simulink model "TorqueVect"  (R2022a)
settings: Solver=VariableStepAuto  StartTime=0.0  StopTime=32  RelTol=1e-3
PreLoadFcn:
  | run('Parameters\FSE_Parameters.m')
undefined symbols (not defined in the file): BRegenEnabledButton, canChannel, CyalphaLookUp, efficiency, Fz_curve, Fz_scaling_long, gearR, izz, jw, Kd, kd, Ki, ki, Kp, kp, l_f, l_r, lambda, m, Mz_max, N, N_lat, N_long, P_max, pid_kd_lat, pid_kd_long, pid_ki_lat, pid_ki_long, pid_kp_lat, pid_kp_long, R_max, rw, steerR, T_i_max, TC_Decr_Gas, TC_Derivative, TC_Incr_Gas, TC_On, TC_Relay_Off, TC_Relay_On, tireCornerStiffness, Ts, TV_On, TV_Override, velocity_lookup, velocity_lookup_lat, y_ref, yrr_scaling
libraries: simulink x218, slpidlib x135, CarMaker4SL x101, TractionControlLibrary x13, canmsglib x9, canlib x8, TorqueVectoringLibrary x6, simulink_extras x4, PedalConversionLibrary x3, PowerControlLibrary x1
(part 18 of 26)

== system TorqueVect/CarMaker/IPG Vehicle/PowerTrain/PTControl Example/PTControl_ALL_CTRL_VC_REGEN/Subsystem1/PowerControl1/PID ==
  PError : Inport
  P_PC : Inport  Port=2
  D_PC : Inport  Port=3
  I_PC : Inport  Port=4
  ResetPID_PC : Inport  Port=5
  PID Controller : slpidlib/PID Controller  Controller=PID  Form=Parallel  TimeDomain=Discrete-time  UseExternalTs=off  SampleTime=0.005  IntegratorMethod=Backward Euler  FilterMethod=Forward Euler  ControllerParametersSource=external  P=1  I=1  UseKiTs=on  D=0  N=100  UseFilter=off  TunerSelectOption=Transfer Function Based (PID Tuner App)  InitialConditionSource=internal  InitialConditionForIntegrator=0  InitialConditionForFilter=0  DifferentiatorICPrevScaledInput=0  ExternalReset=rising  TrackingMode=off  Kt=1  LimitOutput=on  SatLimitsSource=internal  UpperSaturationLimit=80000  LowerSaturationLimit=0  LinearizeAsGain=on  AntiWindupMode=clamping  Kb=2  SaturateOnIntegerOverflow=on  POutMin=[]  POutMax=[]  IOutMin=[]  IOutMax=[]  DOutMin=[]  DOutMax=[]  NOutMin=[]  NOutMax=[]  SumOutMin=[]  SumOutMax=[]  SaturationOutMin=[]  SaturationOutMax=[]  PParamMin=[]  PParamMax=[]  IParamMin=[]  IParamMax=[]  DParamMin=[]  DParamMax=[]  NParamMin=[]  NParamMax=[]  KbParamMin=[]  KbParamMax=[]  KtParamMin=[]  KtParamMax=[]  KbOutMin=[]  KbOutMax=[]  KtOutMin=[]  KtOutMax=[]  IntegratorOutMin=[]  IntegratorOutMax=[]  FilterOutMin=[]  FilterOutMax=[]  SumI1OutMin=[]  SumI1OutMax=[]  SumI2OutMin=[]  SumI2OutMax=[]  SumI3OutMin=[]  SumI3OutMax=[]  SumI4OutMin=[]  SumI4OutMax=[]  SumDOutMin=[]  SumDOutMax=[]  DifferentiatorOutMin=[]  DifferentiatorOutMax=[]  FilterDiffOutCoefMin=[]  FilterDiffOutCoefMax=[]  ReciprocalOutMin=[]  ReciprocalOutMax=[]  SumDenOutMin=[]  SumDenOutMax=[]  SumNumOutMin=[]  SumNumOutMax=[]  DivideOutMin=[]  DivideOutMax=[]  UdiffTsProdOutMin=[]  UdiffTsProdOutMax=[]  NTsProdOutMin=[]  NTsProdOutMax=[]  UintegralTsProdOutMin=[]  UintegralTsProdOutMax=[]  UngainTsProdOutMin=[]  UngainTsProdOutMax=[]  ClampingZeroOutDataTypeStr=Inherit: Inherit via back propagation  ClampingZeroOutMin=[]  ClampingZeroOutMax=[]  FilterDenConstantOutDataTypeStr=Inherit: Inherit via back propagation  FilterDenConstantOutMin=[]  FilterDenConstantOutMax=[]  PCopyOutDataTypeStr=Inherit: Inherit via back propagation  PCopyOutMin=[]  PCopyOutMax=[]  NCopyOutDataTypeStr=Inherit: Inherit via back propagation  NCopyOutMin=[]  NCopyOutMax=[]  IntegratorContinuousStateAttributes=''  IntegratorStateMustResolveToSignalObject=off  IntegratorRTWStateStorageClass=Auto  FilterContinuousStateAttributes=''  FilterStateMustResolveToSignalObject=off  FilterRTWStateStorageClass=Auto  ParallelPVariant=ExternalParameters  IdealPVariant=Disabled  IVariant=ExternalParameters  DVariant=ExternalParameters  IntegratorVariant=Discrete  SatVariant=Enabled  AWVariant=DiscClampingParallel  PCopyVariant=Disabled  TRVariant=Disabled  FdbkBlocksVariant=Feedback  IdealPFdbkVariant=Passthrough  SatFdbkVariant=Passthrough  DerivativeFilterVariant=Differentiator  NVariant=Passthrough  NCopyVariant=Disabled_SignalSpec  FilterICVariant=InternalICsDifferentiator  IntegratorICVariant=InternalICs  ExternalResetVariant=ExternalReset  TRSumVariant=Passthrough  SumFdbkVariant=Enabled  SumVariant=Sum_PID  TsampFilterVariant=InternalTs  TsampNgainVariant=Passthrough  TsampIntegralVariant=Passthrough  ExternalSaturationOutDataTypeStr=Inherit: Same as second input  aMode=0
  PReductionTotal : Outport
  wires:
  PID Controller/1 -> PReductionTotal/1  "control input delta_P"
  D_PC/1 -> PID Controller/4
  P_PC/1 -> PID Controller/2
  PError/1 -> PID Controller/1
  I_PC/1 -> PID Controller/3
  ResetPID_PC/1 -> PID Controller/5

== system TorqueVect/CarMaker/IPG Vehicle/PowerTrain/PTControl Example/PTControl_ALL_CTRL_VC_REGEN/Subsystem1/PowerControl1/PowerError ==
  PPositiveTotal : Inport  Unit=W  PortDimensions=1
      settings: AttributesFormatString=%<Unit>
  FF_PC : Inport  Port=2
  PLimit : Inport  Port=3  OutMin=0  OutMax=80000  Unit=W  PortDimensions=1
      settings: AttributesFormatString=[%<OutMin>, %<OutMax>] %<Unit>
  Product5 : Product
  Saturation2 : Saturate  UpperLimit=250000  LowerLimit=0
      settings: AttributesFormatString=[%<LowerLimit>, %<UpperLimit>] W
  Subtract2 : Sum  Inputs=+-
  PError : Outport  Unit=W  PortDimensions=1
      settings: AttributesFormatString=%<Unit>
  wires:
  FF_PC/1 -> Product5/2
  Subtract2/1 -> Saturation2/1
  PLimit/1 -> Subtract2/2
  PPositiveTotal/1 -> Product5/1
  Saturation2/1 -> PError/1  "power error"
  Product5/1 -> Subtract2/1

== system TorqueVect/CarMaker/IPG Vehicle/PowerTrain/PTControl Example/PTControl_ALL_CTRL_VC_REGEN/Subsystem1/PowerControl1/ResetPID_PC ==
  rThrottlePedal : Inport
  PReductionTotal : Inport  Port=2
  AND : Logic  IconShape=distinctive  AllPortsSameDT=off  OutDataTypeStr=boolean
  AND1 : Logic  Inputs=3  IconShape=distinctive  AllPortsSameDT=off  OutDataTypeStr=boolean
  Compare To Constant1 : simulink/Logic and Bit Operations/Compare To Constant  relop=<=  const=0.1  OutDataTypeStr=boolean
  Compare To Constant2 : simulink/Logic and Bit Operations/Compare To Constant  relop=<=  const=0.15  OutDataTypeStr=boolean
  Compare To Constant3 : simulink/Logic and Bit Operations/Compare To Constant  relop=>=  const=0.09  OutDataTypeStr=boolean
  Compare To Constant4 : simulink/Logic and Bit Operations/Compare To Constant  relop=>  const=0  OutDataTypeStr=boolean
  Detect Fall Negative1 : simulink/Logic and Bit Operations/Detect Fall Negative  vinit=0  OutDataTypeStr=boolean
      settings: SourceProductBaseCode=SL
  Discrete Derivative1 : simulink/Discrete/Discrete Derivative  gainval=1.0  ICPrevScaledInput=0.0  OutMin=[]  OutMax=[]  OutDataType=fixdt(1, 16)  OutScaling=2^-10  DoSatur=off
  OR : Logic  Operator=OR  IconShape=distinctive  AllPortsSameDT=off  OutDataTypeStr=boolean
  ResetPID_PC : Outport
  wires:
  rThrottlePedal/1 -> Compare To Constant1/1, Compare To Constant3/1, Compare To Constant2/1, Discrete Derivative1/1
  Discrete Derivative1/1 -> Detect Fall Negative1/1
  Detect Fall Negative1/1 -> AND1/2  "accel_pedal_falling_or"
  Compare To Constant2/1 -> AND1/1
  Compare To Constant3/1 -> AND1/3
  OR/1 -> ResetPID_PC/1
  AND1/1 -> OR/1
  AND/1 -> OR/2
  Compare To Constant1/1 -> AND/1
  Compare To Constant4/1 -> AND/2
  PReductionTotal/1 -> Compare To Constant4/1

== system TorqueVect/CarMaker/IPG Vehicle/PowerTrain/PTControl Example/PTControl_ALL_CTRL_VC_REGEN/Subsystem1/PowerControl1/Subsystem ==
  PReductionTotal : Inport
  rSplitF : Inport  Port=2
  Product : Product
  Sum : Sum  Inputs=|+-
  PReductionR : Outport
  PReductionF : Outport  Port=2
  wires:
  rSplitF/1 -> Product/2
  PReductionTotal/1 -> Sum/1, Product/1
  Product/1 -> PReductionF/1, Sum/2
  Sum/1 -> PReductionR/1

== system TorqueVect/CarMaker/IPG Vehicle/PowerTrain/PTControl Example/PTControl_ALL_CTRL_VC_REGEN/Subsystem1/PowerControl1/TotalPower ==
  MMotorFL : Inport  OutMin=-42  OutMax=42  Unit=N*m  PortDimensions=1
      settings: AttributesFormatString=[%<OutMin>, %<OutMax>] %<Unit>
  nMotorFL : Inport  Port=2  OutMin=-3000  OutMax=3000  Unit=rad/s  PortDimensions=1
      settings: AttributesFormatString=[%<OutMin>, %<OutMax>] %<Unit>
  MMotorFR : Inport  Port=3  OutMin=-42  OutMax=42  Unit=N*m  PortDimensions=1
      settings: AttributesFormatString=[%<OutMin>, %<OutMax>] %<Unit>
  nMotorFR : Inport  Port=4  OutMin=-3000  OutMax=3000  Unit=rad/s  PortDimensions=1
      settings: AttributesFormatString=[%<OutMin>, %<OutMax>] %<Unit>
  MMotorRL : Inport  Port=5  OutMin=-42  OutMax=42  Unit=N*m  PortDimensions=1
      settings: AttributesFormatString=[%<OutMin>, %<OutMax>] %<Unit>
  nMotorRL : Inport  Port=6  OutMin=-3000  OutMax=3000  Unit=rad/s  PortDimensions=1
      settings: AttributesFormatString=[%<OutMin>, %<OutMax>] %<Unit>
  MMotorRR : Inport  Port=7  OutMin=-42  OutMax=42  Unit=N*m  PortDimensions=1
      settings: AttributesFormatString=[%<OutMin>, %<OutMax>] %<Unit>
  nMotorRR : Inport  Port=8  OutMin=-3000  OutMax=3000  Unit=rad/s  PortDimensions=1
      settings: AttributesFormatString=[%<OutMin>, %<OutMax>] %<Unit>
  PMeasured : Inport  Port=9  OutMin=-250000  OutMax=250000  Unit=W  PortDimensions=1
      settings: AttributesFormatString=[%<OutMin>, %<OutMax>] %<Unit>
  BMeasuredEnable : Inport  Port=10  OutMin=0  OutMax=1  PortDimensions=1
      settings: AttributesFormatString=[%<OutMin> / %<OutMax>]
  Product{2,7..9} (4 alike) : Product
  Saturation{1,3..5} (4 alike) : Saturate  UpperLimit=250000  LowerLimit=0
  Sum1 : Sum  Inputs=++++
  Sum3 : Sum  Inputs=++++
  Switch : Switch  Threshold=1  SaturateOnIntegerOverflow=off  InputSameDT=off
  Switch3 : Switch  Threshold=1  SaturateOnIntegerOverflow=off  InputSameDT=off
  Terminator : Terminator
  PPositiveTotal : Outport  OutMin=0  OutMax=250000  Unit=W  PortDimensions=1
      settings: AttributesFormatString=[%<OutMin>, %<OutMax>] %<Unit>
  wires:
  MMotorRR/1 -> Product9/2
  nMotorRR/1 -> Product9/1
  nMotorRL/1 -> Product8/2
  MMotorRL/1 -> Product8/1
  nMotorFR/1 -> Product7/2
  MMotorFR/1 -> Product7/1
  nMotorFL/1 -> Product2/2
  MMotorFL/1 -> Product2/1
  Product9/1 -> Saturation5/1, Sum1/4
  Product8/1 -> Saturation4/1, Sum1/3
  Product7/1 -> Saturation3/1, Sum1/2
  BMeasuredEnable/1 -> Switch/2, Switch3/2
  Switch3/1 -> Terminator/1
  PMeasured/1 -> Switch/1, Switch3/1
  Switch/1 -> PPositiveTotal/1
  Sum1/1 -> Switch3/3  "tot_powerrrr_RC"
  Saturation1/1 -> Sum3/1
  Saturation4/1 -> Sum3/3
  Product2/1 -> Saturation1/1, Sum1/1
  Saturation5/1 -> Sum3/4
  Sum3/1 -> Switch/3  "tot_powerrrr_PC"
  Saturation3/1 -> Sum3/2

== system TorqueVect/CarMaker/IPG Vehicle/PowerTrain/PTControl Example/PTControl_ALL_CTRL_VC_REGEN/Subsystem1/PowerControl1/WheelTorqueOut ==
  PReductionF : Inport
  PReductionR : Inport  Port=2
  nMotorFL : Inport  Port=3
  nMotorFR : Inport  Port=4
  nMotorRL : Inport  Port=5
  nMotorRR : Inport  Port=6
  Divide{1..4} (4 alike) : Product  Inputs=*/
  Gain : Gain  Gain=0.5
  Gain1 : Gain  Gain=0.5
  Saturation{,5..7} (4 alike) : Saturate  UpperLimit=42  LowerLimit=-42
  Saturation{1..4} (4 alike) : Saturate  UpperLimit=30000  LowerLimit=eps
  MReductionMotorFL : Outport
  MReductionMotorFR : Outport  Port=2
  MReductionMotorRL : Outport  Port=3
  MReductionMotorRR : Outport  Port=4
  wires:
  Divide4/1 -> Saturation7/1
  Divide3/1 -> Saturation6/1
  Divide2/1 -> Saturation5/1
  Divide1/1 -> Saturation/1
  Saturation4/1 -> Divide4/2
  Saturation3/1 -> Divide3/2
  nMotorRR/1 -> Saturation4/1
  nMotorRL/1 -> Saturation3/1
  Gain1/1 -> Divide3/1, Divide4/1
  Saturation2/1 -> Divide2/2
  Saturation1/1 -> Divide1/2
  nMotorFR/1 -> Saturation2/1
  nMotorFL/1 -> Saturation1/1
  Gain/1 -> Divide1/1, Divide2/1
  PReductionR/1 -> Gain1/1
  PReductionF/1 -> Gain/1
  Saturation/1 -> MReductionMotorFL/1
  Saturation5/1 -> MReductionMotorFR/1
  Saturation6/1 -> MReductionMotorRL/1
  Saturation7/1 -> MReductionMotorRR/1

== system TorqueVect/CarMaker/IPG Vehicle/PowerTrain/PTControl Example/PTControl_ALL_CTRL_VC_REGEN/Subsystem1/TC/Slip Ratio Measurement ==
  vLong1 : Inport  Unit=m/s
      settings: AttributesFormatString=%<Unit>
  nMotorFL : Inport  Port=2  Unit=rad/s  PortDimensions=1
      settings: AttributesFormatString=%<Unit>
  nMotorFR : Inport  Port=3  Unit=rad/s  PortDimensions=1
      settings: AttributesFormatString=%<Unit>
  nMotorRL : Inport  Port=4  Unit=rad/s  PortDimensions=1
      settings: AttributesFormatString=%<Unit>
  nMotorRR : Inport  Port=5  Unit=rad/s  PortDimensions=1
      settings: AttributesFormatString=%<Unit>
  aSteerFL : Inport  Port=6
  aSteerFR : Inport  Port=7
  nYaw : Inport  Port=8
  Add : Sum  Inputs=+-
  Add1 : Sum
  Add2 : Sum  Inputs=-+
  Constant : Constant  Value=[0 0 0 0]
  Constant3 : Constant
  Cos : Trigonometry  Operator=cos
  Cos1 : Trigonometry  Operator=cos
  Demux : Demux
  Demux1 : Demux
  Divide : Product  Inputs=/*
  Divide1 : Product  Inputs=*/
  Divide2 : Product  Inputs=/*
  Gain : Gain  Gain=0.1975/13.39
  Mux : Mux
  Mux1 : Mux
  Product : Product
  Saturation : Saturate  UpperLimit=60  LowerLimit=eps
  Saturation1 : Saturate  UpperLimit=1  LowerLimit=0
  Switch1 : Switch  Criteria=u2 > Threshold  Threshold=0.25  SaturateOnIntegerOverflow=off  InputSameDT=off
  halfTrackWidth : Constant  Value=0.5588
  vLong1_1 : InportShadow  Unit=m/s
      settings: AttributesFormatString=%<Unit>
  rSlipMeasuredFL : Outport
  rSlipMeasuredFR : Outport  Port=2
  rSlipMeasuredRL : Outport  Port=3
  rSlipMeasuredRR : Outport  Port=4
  debug : Outport  Port=5
  wires:
  vLong1_1/1 -> Switch1/2
  Add/1 -> Mux1/3, Divide/2  "vWheelFromCarLongRL"
  nMotorFR/1 -> Mux/2
  halfTrackWidth/1 -> Product/2
  Mux1/1 -> Saturation/1
  vLong1/1 -> Add/1, Add1/1
  Demux1/4 -> rSlipMeasuredRR/1
  nYaw/1 -> Product/1
  Saturation1/1 -> Demux1/1
  nMotorRL/1 -> Mux/3
  Demux1/3 -> rSlipMeasuredRL/1
  Gain/1 -> Divide2/2  "m/s"
  Product/1 -> Add1/2, Add/2
  Add1/1 -> Mux1/4, Divide1/1  "vWheelFromCarLongRR"
  nMotorFL/1 -> Mux/1
  Saturation/1 -> Divide2/1
  Cos1/1 -> Divide1/2
  nMotorRR/1 -> Mux/4
  Divide1/1 -> Mux1/2  "vWheelFromCarLongFR"
  Demux1/1 -> rSlipMeasuredFL/1
  Mux/1 -> Gain/1  "omega"
  Switch1/1 -> Saturation1/1
  Cos/1 -> Divide/1
  Constant/1 -> Switch1/3
  Divide/1 -> Mux1/1  "vWheelFromCarLongFL"
  Demux1/2 -> rSlipMeasuredFR/1
  aSteerFR/1 -> Cos1/1
  aSteerFL/1 -> Cos/1
  Divide2/1 -> Add2/2
  Constant3/1 -> Add2/1
  Add2/1 -> Demux/1, Switch1/1
  Demux/1 -> debug/1

== system TorqueVect/CarMaker/IPG Vehicle/PowerTrain/PTControl Example/PTControl_ALL_CTRL_VC_REGEN/Subsystem1/TC/TractionControlFL ==
  rSlipTarget : Inport
  rSlipMeasured : Inport  Port=2
  BEnableTC : Inport  Port=3
  P_TC : Inport  Port=4
  D_TC : Inport  Port=5
  I_TC : Inport  Port=6
  FF_TC : Inport  Port=7
  MMotorMax : Inport  Port=8
  MMotorRequest : Inport  Port=9
  resetTC : Inport  Port=10
  If : If  NumInputs=2  IfExpression=u1 <= 0  ElseIfExpressions=u2 > u1
  If Action Subsystem : Subsystem  TreatAsAtomicUnit=on
  If Action Subsystem1 : Subsystem  TreatAsAtomicUnit=on
  If Action Subsystem2 : Subsystem  TreatAsAtomicUnit=on
  Merge : Merge  Inputs=3
  PID Controller : Subsystem  TreatAsAtomicUnit=on
  Product : Product
  Product1 : Product
  Saturation : Saturate  UpperLimit=1  LowerLimit=0
  Saturation1 : Saturate  UpperLimit=21  LowerLimit=0
  Sum1 : Sum  Inputs=|-+
  MMotorDemanded : Outport  VectorParamsAs1DForOutWhenUnconnected=off
  wires:
  rSlipTarget/1 -> Sum1/1
  MMotorRequest/1 -> If Action Subsystem/1(MMotorRequest), If/1, If Action Subsystem2/1(MMotorRequest)
  Saturation1/1 -> If Action Subsystem2/2(In2), If/2
  If/2 -> If Action Subsystem1/Action
  P_TC/1 -> PID Controller/3(Kp_TC)
  If Action Subsystem2/1(Out1) -> Merge/3
  FF_TC/1 -> Product/2
  Product/1 -> Sum1/2
  D_TC/1 -> PID Controller/4(Kd_TC)
  Saturation/1 -> PID Controller/1(rSlipError)
  If Action Subsystem/1(Out1) -> Merge/1
  Product1/1 -> Saturation/1
  If/3 -> If Action Subsystem2/Action
  BEnableTC/1 -> Product1/2, PID Controller/2(BEnable_TC)
  If Action Subsystem1/1(Out1) -> Merge/2
  PID Controller/1(MMotorReduction) -> Saturation1/1
  I_TC/1 -> PID Controller/5(Ki_TC)
  Merge/1 -> MMotorDemanded/1
  Sum1/1 -> Product1/1
  If/1 -> If Action Subsystem/Action
  rSlipMeasured/1 -> Product/1
  MMotorMax/1 -> PID Controller/6(MMotorMax)
  resetTC/1 -> PID Controller/7(resetTC)

== system TorqueVect/CarMaker/IPG Vehicle/PowerTrain/PTControl Example/PTControl_ALL_CTRL_VC_REGEN/Subsystem1/TC/TractionControlFR ==
  rSlipTarget : Inport
  rSlipMeasured : Inport  Port=2
  BEnableTC : Inport  Port=3
  P_TC : Inport  Port=4
  D_TC : Inport  Port=5
  I_TC : Inport  Port=6
  FF_TC : Inport  Port=7
  MMotorMax : Inport  Port=8
  MMotorRequest : Inport  Port=9
  resetTC : Inport  Port=10
  If : If  NumInputs=2  IfExpression=u1 <= 0  ElseIfExpressions=u2 > u1
  If Action Subsystem : Subsystem  TreatAsAtomicUnit=on
  If Action Subsystem1 : Subsystem  TreatAsAtomicUnit=on
  If Action Subsystem2 : Subsystem  TreatAsAtomicUnit=on
  Merge : Merge  Inputs=3
  PID Controller : Subsystem  TreatAsAtomicUnit=on
  Product : Product
  Product1 : Product
  Saturation : Saturate  UpperLimit=1  LowerLimit=0
  Saturation1 : Saturate  UpperLimit=21  LowerLimit=0
  Sum1 : Sum  Inputs=|-+
  MMotorDemanded : Outport  VectorParamsAs1DForOutWhenUnconnected=off
  wires:
  rSlipTarget/1 -> Sum1/1
  MMotorRequest/1 -> If Action Subsystem/1(MMotorRequest), If/1, If Action Subsystem2/1(MMotorRequest)
  Saturation1/1 -> If Action Subsystem2/2(In2), If/2
  If/2 -> If Action Subsystem1/Action
  P_TC/1 -> PID Controller/3(Kp_TC)
  If Action Subsystem2/1(Out1) -> Merge/3
  FF_TC/1 -> Product/2
  Product/1 -> Sum1/2
  D_TC/1 -> PID Controller/4(Kd_TC)
  Saturation/1 -> PID Controller/1(rSlipError)
  If Action Subsystem/1(Out1) -> Merge/1
  Product1/1 -> Saturation/1
  If/3 -> If Action Subsystem2/Action
  BEnableTC/1 -> Product1/2, PID Controller/2(BEnable_TC)
  If Action Subsystem1/1(Out1) -> Merge/2
  PID Controller/1(MMotorReduction) -> Saturation1/1
  I_TC/1 -> PID Controller/5(Ki_TC)
  Merge/1 -> MMotorDemanded/1
  Sum1/1 -> Product1/1
  If/1 -> If Action Subsystem/Action
  rSlipMeasured/1 -> Product/1
  MMotorMax/1 -> PID Controller/6(MMotorMax)
  resetTC/1 -> PID Controller/7(resetTC)

== system TorqueVect/CarMaker/IPG Vehicle/PowerTrain/PTControl Example/PTControl_ALL_CTRL_VC_REGEN/Subsystem1/TC/TractionControlRL ==
  rSlipTarget : Inport
  rSlipMeasured : Inport  Port=2
  BEnableTC : Inport  Port=3
  P_TC : Inport  Port=4
  D_TC : Inport  Port=5
  I_TC : Inport  Port=6
  FF_TC : Inport  Port=7
  MMotorMax : Inport  Port=8
  MMotorRequest : Inport  Port=9
  resetTC : Inport  Port=10
  If : If  NumInputs=2  IfExpression=u1 <= 0  ElseIfExpressions=u2 > u1
  If Action Subsystem : Subsystem  TreatAsAtomicUnit=on
  If Action Subsystem1 : Subsystem  TreatAsAtomicUnit=on
  If Action Subsystem2 : Subsystem  TreatAsAtomicUnit=on
  Merge : Merge  Inputs=3
  PID Controller : Subsystem  TreatAsAtomicUnit=on
  Product : Product
  Product1 : Product
  Saturation : Saturate  UpperLimit=1  LowerLimit=0
  Saturation1 : Saturate  UpperLimit=21  LowerLimit=0
  Sum1 : Sum  Inputs=|-+
  MMotorDemanded : Outport  VectorParamsAs1DForOutWhenUnconnected=off
  wires:
  rSlipTarget/1 -> Sum1/1
  MMotorRequest/1 -> If Action Subsystem/1(MMotorRequest), If/1, If Action Subsystem2/1(MMotorRequest)
  Saturation1/1 -> If Action Subsystem2/2(In2), If/2
  If/2 -> If Action Subsystem1/Action
  P_TC/1 -> PID Controller/3(Kp_TC)
  If Action Subsystem2/1(Out1) -> Merge/3
  FF_TC/1 -> Product/2
  Product/1 -> Sum1/2
  D_TC/1 -> PID Controller/4(Kd_TC)
  Saturation/1 -> PID Controller/1(rSlipError)
  If Action Subsystem/1(Out1) -> Merge/1
  Product1/1 -> Saturation/1
  If/3 -> If Action Subsystem2/Action
  BEnableTC/1 -> Product1/2, PID Controller/2(BEnable_TC)
  If Action Subsystem1/1(Out1) -> Merge/2
  PID Controller/1(MMotorReduction) -> Saturation1/1
  I_TC/1 -> PID Controller/5(Ki_TC)
  Merge/1 -> MMotorDemanded/1
  Sum1/1 -> Product1/1
  If/1 -> If Action Subsystem/Action
  rSlipMeasured/1 -> Product/1
  MMotorMax/1 -> PID Controller/6(MMotorMax)
  resetTC/1 -> PID Controller/7(resetTC)

== system TorqueVect/CarMaker/IPG Vehicle/PowerTrain/PTControl Example/PTControl_ALL_CTRL_VC_REGEN/Subsystem1/TC/TractionControlRR ==
  rSlipTarget : Inport
  rSlipMeasured : Inport  Port=2
  BEnableTC : Inport  Port=3
  P_TC : Inport  Port=4
  D_TC : Inport  Port=5
  I_TC : Inport  Port=6
  FF_TC : Inport  Port=7
  MMotorMax : Inport  Port=8
  MMotorRequest : Inport  Port=9
  resetTC : Inport  Port=10
  If : If  NumInputs=2  IfExpression=u1 <= 0  ElseIfExpressions=u2 > u1
  If Action Subsystem : Subsystem  TreatAsAtomicUnit=on
  If Action Subsystem1 : Subsystem  TreatAsAtomicUnit=on
  If Action Subsystem2 : Subsystem  TreatAsAtomicUnit=on
  Merge : Merge  Inputs=3
  PID Controller : Subsystem  TreatAsAtomicUnit=on
  Product : Product
  Product1 : Product
  Saturation : Saturate  UpperLimit=1  LowerLimit=0
  Saturation1 : Saturate  UpperLimit=21  LowerLimit=0
  Sum1 : Sum  Inputs=|-+
  MMotorDemanded : Outport  VectorParamsAs1DForOutWhenUnconnected=off
  wires:
  rSlipTarget/1 -> Sum1/1
  MMotorRequest/1 -> If Action Subsystem/1(MMotorRequest), If/1, If Action Subsystem2/1(MMotorRequest)
  Saturation1/1 -> If Action Subsystem2/2(In2), If/2
  If/2 -> If Action Subsystem1/Action
  P_TC/1 -> PID Controller/3(Kp_TC)
  If Action Subsystem2/1(Out1) -> Merge/3
  FF_TC/1 -> Product/2
  Product/1 -> Sum1/2
  D_TC/1 -> PID Controller/4(Kd_TC)
  Saturation/1 -> PID Controller/1(rSlipError)
  If Action Subsystem/1(Out1) -> Merge/1
  Product1/1 -> Saturation/1
  If/3 -> If Action Subsystem2/Action
  BEnableTC/1 -> PID Controller/2(BEnable_TC), Product1/2
  If Action Subsystem1/1(Out1) -> Merge/2
  PID Controller/1(MMotorReduction) -> Saturation1/1
  I_TC/1 -> PID Controller/5(Ki_TC)
  Merge/1 -> MMotorDemanded/1
  Sum1/1 -> Product1/1
  If/1 -> If Action Subsystem/Action
  rSlipMeasured/1 -> Product/1
  MMotorMax/1 -> PID Controller/6(MMotorMax)
  resetTC/1 -> PID Controller/7(resetTC)

== system TorqueVect/CarMaker/IPG Vehicle/PowerTrain/PTControl Example/PTControl_ALL_CTRL_VC_REGEN/Subsystem1/Torque Modification/Torque Limit Check FL ==
  note: Checks for max value below 0 Nm when RC is acting
  note: Checks for min value when PC is acting
  MTorqueNewFL : Inport
  MDemandMotorFL : Inport  Port=2
  Max : MinMax  Function=max  Inputs=2
  Min : MinMax  Inputs=2
  Saturation : Saturate  UpperLimit=0  LowerLimit=-21
  Saturation1 : Saturate  UpperLimit=21  LowerLimit=0
  Switch : Switch  Criteria=u2 > Threshold  SaturateOnIntegerOverflow=off  InputSameDT=off
  MTorqueModFL : Outport
  wires:
  MDemandMotorFL/1 -> [MDemandMotorRL]
  [MDemandMotorRL] -> Min/1
  MTorqueNewFL/1 -> Saturation/1, Saturation1/1
  Switch/1 -> MTorqueModFL/1
  [MDemandMotorRL] -> Switch/2
  Min/1 -> Switch/1
  Max/1 -> Switch/3
  [MDemandMotorRL] -> Max/2
  Saturation/1 -> Max/1
  Saturation1/1 -> Min/2

== system TorqueVect/CarMaker/IPG Vehicle/PowerTrain/PTControl Example/PTControl_ALL_CTRL_VC_REGEN/Subsystem1/Torque Modification/Torque Limit Check FR ==
  note: Checks for max value below 0 Nm when RC is acting
  note: Checks for min value when PC is acting
  MTorqueNewFR : Inport
  MDemandMotorFR : Inport  Port=2
  Max : MinMax  Function=max  Inputs=2
  Min : MinMax  Inputs=2
  Saturation : Saturate  UpperLimit=0  LowerLimit=-21
  Saturation1 : Saturate  UpperLimit=21  LowerLimit=0
  Switch : Switch  Criteria=u2 > Threshold  SaturateOnIntegerOverflow=off  InputSameDT=off
  MTorqueModFR : Outport
  wires:
  MDemandMotorFR/1 -> [MDemandMotorRL]
  [MDemandMotorRL] -> Min/1
  MTorqueNewFR/1 -> Saturation/1, Saturation1/1
  Switch/1 -> MTorqueModFR/1
  [MDemandMotorRL] -> Switch/2
  Min/1 -> Switch/1
  Max/1 -> Switch/3
  [MDemandMotorRL] -> Max/2
  Saturation/1 -> Max/1
  Saturation1/1 -> Min/2

== system TorqueVect/CarMaker/IPG Vehicle/PowerTrain/PTControl Example/PTControl_ALL_CTRL_VC_REGEN/Subsystem1/Torque Modification/Torque Limit Check RL ==
  note: Checks for max value below 0 Nm when RC is acting
  note: Checks for min value when PC is acting
  MTorqueNewRL : Inport
  MDemandMotorRL : Inport  Port=2
  Max : MinMax  Function=max  Inputs=2
  Min : MinMax  Inputs=2
  Saturation : Saturate  UpperLimit=0  LowerLimit=-21
  Saturation1 : Saturate  UpperLimit=21  LowerLimit=0
  Switch : Switch  Criteria=u2 > Threshold  SaturateOnIntegerOverflow=off  InputSameDT=off
  MTorqueModRL : Outport
  wires:
  MDemandMotorRL/1 -> [MDemandMotorRL]
  [MDemandMotorRL] -> Min/1
  MTorqueNewRL/1 -> Saturation/1, Saturation1/1
  Switch/1 -> MTorqueModRL/1
  [MDemandMotorRL] -> Switch/2
  Min/1 -> Switch/1
  Max/1 -> Switch/3
  [MDemandMotorRL] -> Max/2
  Saturation/1 -> Max/1
  Saturation1/1 -> Min/2

== system TorqueVect/CarMaker/IPG Vehicle/PowerTrain/PTControl Example/PTControl_ALL_CTRL_VC_REGEN/Subsystem1/Torque Modification/Torque Limit Check RR ==
  note: Checks for max value below 0 Nm when RC is acting
  note: Checks for min value when PC is acting
  MTorqueNewRR : Inport
  MDemandMotorRR : Inport  Port=2
  Max : MinMax  Function=max  Inputs=2
  Min : MinMax  Inputs=2
  Saturation : Saturate  UpperLimit=0  LowerLimit=-21
  Saturation1 : Saturate  UpperLimit=21  LowerLimit=0
  Switch : Switch  Criteria=u2 > Threshold  SaturateOnIntegerOverflow=off  InputSameDT=off
  MTorqueModRR : Outport
  wires:
  MDemandMotorRR/1 -> [MDemandMotorRL]
  [MDemandMotorRL] -> Min/1
  MTorqueNewRR/1 -> Saturation/1, Saturation1/1
  Switch/1 -> MTorqueModRR/1
  [MDemandMotorRL] -> Switch/2
  Min/1 -> Switch/1
  Max/1 -> Switch/3
  [MDemandMotorRL] -> Max/2
  Saturation/1 -> Max/1
  Saturation1/1 -> Min/2

== system TorqueVect/CarMaker/IPG Vehicle/PowerTrain/PTControl Example/PTControl_ALL_CTRL_VC_REGEN/Subsystem1/Torque Vectoring/F PID ==
  BEnable : Inport
  NTorqueMaxDelta : Inport  Port=2
  NTorqueMax : Inport  Port=3
  NTorqueAxle : Inport  Port=4
  aSlip : Inport  Port=5
  P_YR : Inport  Port=6
  D_YR : Inport  Port=7
  I_YR : Inport  Port=8
  NBrake : Inport  Port=9
  Abs : Abs  SaturateOnIntegerOverflow=off
  Abs2 : Abs  SaturateOnIntegerOverflow=off
  Add : Sum  Inputs=+-
  Gain : Gain  Gain=0.5
  Gain1 : Gain  Gain=-1
  If : If  IfExpression=u1 < 0.4
  If Action Subsystem : Subsystem  TreatAsAtomicUnit=on
  If Action Subsystem1 : Subsystem  TreatAsAtomicUnit=on
  Min : MinMax  Inputs=3
  PID Controller : slpidlib/PID Controller  Controller=PID  Form=Ideal  TimeDomain=Discrete-time  UseExternalTs=off  SampleTime=0.005  IntegratorMethod=Forward Euler  FilterMethod=Forward Euler  ControllerParametersSource=external  P=1  I=1  UseKiTs=on  D=0  N=100  UseFilter=off  TunerSelectOption=Transfer Function Based (PID Tuner App)  InitialConditionSource=internal  InitialConditionForIntegrator=0  InitialConditionForFilter=0  DifferentiatorICPrevScaledInput=0  ExternalReset=either  TrackingMode=off  Kt=1  LimitOutput=off  SatLimitsSource=external  UpperSaturationLimit=inf  LowerSaturationLimit=-inf  LinearizeAsGain=on  AntiWindupMode=clamping  Kb=1  POutMin=[]  POutMax=[]  IOutMin=[]  IOutMax=[]  DOutMin=[]  DOutMax=[]  NOutMin=[]  NOutMax=[]  SumOutMin=[]  SumOutMax=[]  SaturationOutMin=[]  SaturationOutMax=[]  PParamMin=[]  PParamMax=[]  IParamMin=[]  IParamMax=[]  DParamMin=[]  DParamMax=[]  NParamMin=[]  NParamMax=[]  KbParamMin=[]  KbParamMax=[]  KtParamMin=[]  KtParamMax=[]  KbOutMin=[]  KbOutMax=[]  KtOutMin=[]  KtOutMax=[]  IntegratorOutMin=[]  IntegratorOutMax=[]  FilterOutMin=[]  FilterOutMax=[]  SumI1OutMin=[]  SumI1OutMax=[]  SumI2OutMin=[]  SumI2OutMax=[]  SumI3OutMin=[]  SumI3OutMax=[]  SumI4OutMin=[]  SumI4OutMax=[]  SumDOutMin=[]  SumDOutMax=[]  DifferentiatorOutMin=[]  DifferentiatorOutMax=[]  FilterDiffOutCoefMin=[]  FilterDiffOutCoefMax=[]  ReciprocalOutMin=[]  ReciprocalOutMax=[]  SumDenOutMin=[]  SumDenOutMax=[]  SumNumOutMin=[]  SumNumOutMax=[]  DivideOutMin=[]  DivideOutMax=[]  UdiffTsProdOutMin=[]  UdiffTsProdOutMax=[]  NTsProdOutMin=[]  NTsProdOutMax=[]  UintegralTsProdOutMin=[]  UintegralTsProdOutMax=[]  UngainTsProdOutMin=[]  UngainTsProdOutMax=[]  ClampingZeroOutDataTypeStr=Inherit: Inherit via back propagation  ClampingZeroOutMin=[]  ClampingZeroOutMax=[]  FilterDenConstantOutDataTypeStr=Inherit: Inherit via back propagation  FilterDenConstantOutMin=[]  FilterDenConstantOutMax=[]  PCopyOutDataTypeStr=Inherit: Inherit via back propagation  PCopyOutMin=[]  PCopyOutMax=[]  NCopyOutDataTypeStr=Inherit: Inherit via back propagation  NCopyOutMin=[]  NCopyOutMax=[]  IntegratorContinuousStateAttributes=''  IntegratorStateMustResolveToSignalObject=off  IntegratorRTWStateStorageClass=Auto  FilterContinuousStateAttributes=''  FilterStateMustResolveToSignalObject=off  FilterRTWStateStorageClass=Auto  ParallelPVariant=Passthrough  IdealPVariant=ExternalParameters  IVariant=ExternalParameters  DVariant=ExternalParameters  IntegratorVariant=Discrete  SatVariant=Disabled  AWVariant=Passthrough  PCopyVariant=Disabled  TRVariant=Disabled  FdbkBlocksVariant=Forward  IdealPFdbkVariant=Disabled  SatFdbkVariant=Disabled  DerivativeFilterVariant=Differentiator  NVariant=Passthrough  NCopyVariant=Disabled_SignalSpec  FilterICVariant=InternalICsDifferentiator  IntegratorICVariant=InternalICs  ExternalResetVariant=ExternalReset  TRSumVariant=Passthrough  SumFdbkVariant=Disabled  SumVariant=Sum_PID  TsampFilterVariant=InternalTs  TsampNgainVariant=Passthrough  TsampIntegralVariant=Passthrough  ExternalSaturationOutDataTypeStr=Inherit: Same as second input  aMode=0
  Product : Product  Inputs=3
  Saturation Dynamic : simulink/Discontinuities/Saturation Dynamic  OutMin=[]  OutMax=[]  OutDataTypeStr=Inherit: Same as second input  OutDataType=fixdt(1, 16)  OutScaling=2^-10  DoSatur=off
  Saturation Dynamic1 : simulink/Discontinuities/Saturation Dynamic  OutMin=[]  OutMax=[]  OutDataTypeStr=Inherit: Same as second input  OutDataType=fixdt(1, 16)  OutScaling=2^-10  DoSatur=off
  Sign : Signum
  Switch : Switch  Threshold=0.4  SaturateOnIntegerOverflow=off  InputSameDT=off
  Switch1 : Switch  Threshold=0.4  SaturateOnIntegerOverflow=off  InputSameDT=off
  NTorqueLeftOut : Outport
  NTorqueRightOut : Outport  Port=2
  wires:
  I_YR/1 -> PID Controller/3
  [NTorqueWheel] -> If Action Subsystem1/1(NTorqueWheel), If Action Subsystem/1(NTorqueWheel)
  aSlip/1 -> PID Controller/1
  Saturation Dynamic1/1 -> NTorqueRightOut/1
  NTorqueMax/1 -> [NTorqueMax]
  [NTorqueWheel] -> Abs/1
  NTorqueAxle/1 -> Gain/1
  [NTorqueMax] -> Add/1
  [BEnable] -> PID Controller/5
  Gain/1 -> [NTorqueWheel]
  NBrake/1 -> If/1, Switch/2, Switch1/2
  P_YR/1 -> PID Controller/2
  [NTorqueMax] -> Saturation Dynamic/1, Saturation Dynamic1/1, Gain1/1
  [BEnable] -> Product/1
  Sign/1 -> Product/3
  [NTorqueTV] -> Abs2/1
  Saturation Dynamic/1 -> NTorqueLeftOut/1
  Abs/1 -> Add/2
  Product/1 -> If Action Subsystem/2(NTorqueDelta)
  Add/1 -> Min/2
  BEnable/1 -> [BEnable]
  Gain1/1 -> Saturation Dynamic/3, Saturation Dynamic1/3
  If/2 -> If Action Subsystem1/Action
  Switch1/1 -> Saturation Dynamic1/2
  If Action Subsystem/1(NTorqueLeftOut) -> Switch/3
  If Action Subsystem1/2(NTorqueRightOut) -> Switch1/1
  PID Controller/1 -> [NTorqueTV]
  [NTorqueTV] -> Sign/1
  If Action Subsystem1/1(NTorqueLeftOut) -> Switch/1
  NTorqueMaxDelta/1 -> Min/1
  Min/1 -> Product/2
  Switch/1 -> Saturation Dynamic/2
  Abs2/1 -> Min/3
  If/1 -> If Action Subsystem/Action
  D_YR/1 -> PID Controller/4
  If Action Subsystem/2(NTorqueRightOut) -> Switch1/3

== system TorqueVect/CarMaker/IPG Vehicle/PowerTrain/PTControl Example/PTControl_ALL_CTRL_VC_REGEN/Subsystem1/Torque Vectoring/R PID ==
  BEnable : Inport
  NTorqueMaxDelta : Inport  Port=2
  NTorqueMax : Inport  Port=3
  NTorqueAxle : Inport  Port=4
  aSlip : Inport  Port=5
  P_YR : Inport  Port=6
  D_YR : Inport  Port=7
  I_YR : Inport  Port=8
  NBrake : Inport  Port=9
  Abs : Abs  SaturateOnIntegerOverflow=off
  Abs2 : Abs  SaturateOnIntegerOverflow=off
  Add : Sum  Inputs=+-
  Gain : Gain  Gain=0.5
  Gain1 : Gain  Gain=-1
  If : If  IfExpression=u1 < 0.4
  If Action Subsystem : Subsystem  TreatAsAtomicUnit=on
  If Action Subsystem1 : Subsystem  TreatAsAtomicUnit=on
  Min : MinMax  Inputs=3
  PID Controller : slpidlib/PID Controller  Controller=PID  Form=Ideal  TimeDomain=Discrete-time  UseExternalTs=off  SampleTime=0.005  IntegratorMethod=Forward Euler  FilterMethod=Forward Euler  ControllerParametersSource=external  P=1  I=1  UseKiTs=on  D=0  N=100  UseFilter=off  TunerSelectOption=Transfer Function Based (PID Tuner App)  InitialConditionSource=internal  InitialConditionForIntegrator=0  InitialConditionForFilter=0  DifferentiatorICPrevScaledInput=0  ExternalReset=either  TrackingMode=off  Kt=1  LimitOutput=off  SatLimitsSource=external  UpperSaturationLimit=inf  LowerSaturationLimit=-inf  LinearizeAsGain=on  AntiWindupMode=clamping  Kb=1  POutMin=[]  POutMax=[]  IOutMin=[]  IOutMax=[]  DOutMin=[]  DOutMax=[]  NOutMin=[]  NOutMax=[]  SumOutMin=[]  SumOutMax=[]  SaturationOutMin=[]  SaturationOutMax=[]  PParamMin=[]  PParamMax=[]  IParamMin=[]  IParamMax=[]  DParamMin=[]  DParamMax=[]  NParamMin=[]  NParamMax=[]  KbParamMin=[]  KbParamMax=[]  KtParamMin=[]  KtParamMax=[]  KbOutMin=[]  KbOutMax=[]  KtOutMin=[]  KtOutMax=[]  IntegratorOutMin=[]  IntegratorOutMax=[]  FilterOutMin=[]  FilterOutMax=[]  SumI1OutMin=[]  SumI1OutMax=[]  SumI2OutMin=[]  SumI2OutMax=[]  SumI3OutMin=[]  SumI3OutMax=[]  SumI4OutMin=[]  SumI4OutMax=[]  SumDOutMin=[]  SumDOutMax=[]  DifferentiatorOutMin=[]  DifferentiatorOutMax=[]  FilterDiffOutCoefMin=[]  FilterDiffOutCoefMax=[]  ReciprocalOutMin=[]  ReciprocalOutMax=[]  SumDenOutMin=[]  SumDenOutMax=[]  SumNumOutMin=[]  SumNumOutMax=[]  DivideOutMin=[]  DivideOutMax=[]  UdiffTsProdOutMin=[]  UdiffTsProdOutMax=[]  NTsProdOutMin=[]  NTsProdOutMax=[]  UintegralTsProdOutMin=[]  UintegralTsProdOutMax=[]  UngainTsProdOutMin=[]  UngainTsProdOutMax=[]  ClampingZeroOutDataTypeStr=Inherit: Inherit via back propagation  ClampingZeroOutMin=[]  ClampingZeroOutMax=[]  FilterDenConstantOutDataTypeStr=Inherit: Inherit via back propagation  FilterDenConstantOutMin=[]  FilterDenConstantOutMax=[]  PCopyOutDataTypeStr=Inherit: Inherit via back propagation  PCopyOutMin=[]  PCopyOutMax=[]  NCopyOutDataTypeStr=Inherit: Inherit via back propagation  NCopyOutMin=[]  NCopyOutMax=[]  IntegratorContinuousStateAttributes=''  IntegratorStateMustResolveToSignalObject=off  IntegratorRTWStateStorageClass=Auto  FilterContinuousStateAttributes=''  FilterStateMustResolveToSignalObject=off  FilterRTWStateStorageClass=Auto  ParallelPVariant=Passthrough  IdealPVariant=ExternalParameters  IVariant=ExternalParameters  DVariant=ExternalParameters  IntegratorVariant=Discrete  SatVariant=Disabled  AWVariant=Passthrough  PCopyVariant=Disabled  TRVariant=Disabled  FdbkBlocksVariant=Forward  IdealPFdbkVariant=Disabled  SatFdbkVariant=Disabled  DerivativeFilterVariant=Differentiator  NVariant=Passthrough  NCopyVariant=Disabled_SignalSpec  FilterICVariant=InternalICsDifferentiator  IntegratorICVariant=InternalICs  ExternalResetVariant=ExternalReset  TRSumVariant=Passthrough  SumFdbkVariant=Disabled  SumVariant=Sum_PID  TsampFilterVariant=InternalTs  TsampNgainVariant=Passthrough  TsampIntegralVariant=Passthrough  ExternalSaturationOutDataTypeStr=Inherit: Same as second input  aMode=0
  Product : Product  Inputs=3
  Saturation Dynamic : simulink/Discontinuities/Saturation Dynamic  OutMin=[]  OutMax=[]  OutDataTypeStr=Inherit: Same as second input  OutDataType=fixdt(1, 16)  OutScaling=2^-10  DoSatur=off
  Saturation Dynamic1 : simulink/Discontinuities/Saturation Dynamic  OutMin=[]  OutMax=[]  OutDataTypeStr=Inherit: Same as second input  OutDataType=fixdt(1, 16)  OutScaling=2^-10  DoSatur=off
  Sign : Signum
  Switch : Switch  Threshold=0.4  SaturateOnIntegerOverflow=off  InputSameDT=off
  Switch1 : Switch  Threshold=0.4  SaturateOnIntegerOverflow=off  InputSameDT=off
  NTorqueLeftOut : Outport
  NTorqueRightOut : Outport  Port=2
  wires:
  I_YR/1 -> PID Controller/3
  [NTorqueWheel] -> If Action Subsystem1/1(NTorqueWheel), If Action Subsystem/1(NTorqueWheel)
  aSlip/1 -> PID Controller/1
  Saturation Dynamic1/1 -> NTorqueRightOut/1
  NTorqueMax/1 -> [NTorqueMax]
  [NTorqueWheel] -> Abs/1
  NTorqueAxle/1 -> Gain/1
  [NTorqueMax] -> Add/1
  [BEnable] -> PID Controller/5
  Gain/1 -> [NTorqueWheel]
  NBrake/1 -> If/1, Switch/2, Switch1/2
  P_YR/1 -> PID Controller/2
  [NTorqueMax] -> Saturation Dynamic/1, Saturation Dynamic1/1, Gain1/1
  [BEnable] -> Product/1
  Sign/1 -> Product/3
  [NTorqueTV] -> Abs2/1
  Saturation Dynamic/1 -> NTorqueLeftOut/1
  Abs/1 -> Add/2
  Product/1 -> If Action Subsystem/2(NTorqueDelta)
  Add/1 -> Min/2
  BEnable/1 -> [BEnable]
  Gain1/1 -> Saturation Dynamic/3, Saturation Dynamic1/3
  If/2 -> If Action Subsystem1/Action
  Switch1/1 -> Saturation Dynamic1/2
  If Action Subsystem/1(NTorqueLeftOut) -> Switch/3
  If Action Subsystem1/2(NTorqueRightOut) -> Switch1/1
  PID Controller/1 -> [NTorqueTV]
  [NTorqueTV] -> Sign/1
  If Action Subsystem1/1(NTorqueLeftOut) -> Switch/1
  NTorqueMaxDelta/1 -> Min/1
  Min/1 -> Product/2
  Switch/1 -> Saturation Dynamic/2
  Abs2/1 -> Min/3
  If/1 -> If Action Subsystem/Action
  D_YR/1 -> PID Controller/4
  If Action Subsystem/2(NTorqueRightOut) -> Switch1/3

== system TorqueVect/CarMaker/IPG Vehicle/PowerTrain/PTControl Example/PTControl_ALL_CTRL_VC_REGEN/Subsystem1/Torque Vectoring/Slip Angle Error Calculation ==
  vLat : Inport  Unit=m/s  PortDimensions=1
      settings: AttributesFormatString=%<Unit>
  vLong : Inport  Port=2  Unit=m/s  PortDimensions=1
      settings: AttributesFormatString=%<Unit>
  aSteerWheel : Inport  Port=3  Unit=rad  PortDimensions=1
      settings: AttributesFormatString=%<Unit>
  rSteerWheel : Inport  Port=4
  Add1 : Sum  Inputs=-+
  Atan : Trigonometry  Operator=atan
  Divide : Product  Inputs=*/
  Gain : Gain  Gain=-1
  Product : Product
  Saturation : Saturate  UpperLimit=60  LowerLimit=eps
  aSlip : Outport  VectorParamsAs1DForOutWhenUnconnected=off
  wires:
  vLat/1 -> Divide/1
  Product/1 -> Add1/2  "Wheel Angle"
  Atan/1 -> Add1/1  "Yaw Angle"
  aSteerWheel/1 -> Product/1
  Divide/1 -> Atan/1
  rSteerWheel/1 -> Product/2
  vLong/1 -> Saturation/1
  Saturation/1 -> Divide/2
  Add1/1 -> Gain/1  "Error"
  Gain/1 -> aSlip/1

== system TorqueVect/CarMaker/IPG Vehicle/PowerTrain/PTControl Example/PTControl_ALL_CTRL_VC_REGEN/Subsystem1/Torque Vectoring/TV Enable Checker ==
  vLong : Inport  Unit=m/s  PortDimensions=1
      settings: AttributesFormatString=%<Unit>
  aSteerWheel : Inport  Port=2  Unit=rad  PortDimensions=1
      settings: AttributesFormatString=%<Unit>
  vLongMin : Inport  Port=3  Unit=m/s  PortDimensions=1
      settings: AttributesFormatString=%<Unit>
  aSteerWheelMin : Inport  Port=4  Unit=rad  PortDimensions=1
      settings: AttributesFormatString=%<Unit>
  BTorqueVectoringEnable : Inport  Port=5
  Abs : Abs  ZeroCross=off  SaturateOnIntegerOverflow=off
  Logical Operator : Logic  Inputs=3  AllPortsSameDT=off  OutDataTypeStr=boolean
  Relational Operator : RelationalOperator  Operator=>  OutDataTypeStr=boolean  RndMeth=Simplest  InputSameDT=off
  Relational Operator1 : RelationalOperator  Operator=>  OutDataTypeStr=boolean  RndMeth=Simplest  InputSameDT=off
  BEnable : Outport  VectorParamsAs1DForOutWhenUnconnected=off
  wires:
  Relational Operator1/1 -> Logical Operator/2
  vLongMin/1 -> Relational Operator/2
  Logical Operator/1 -> BEnable/1
  Relational Operator/1 -> Logical Operator/1
  vLong/1 -> Relational Operator/1
  BTorqueVectoringEnable/1 -> Logical Operator/3
  Abs/1 -> Relational Operator1/1
  aSteerWheelMin/1 -> Relational Operator1/2
  aSteerWheel/1 -> Abs/1

== system TorqueVect/CarMaker/IPG Vehicle/PowerTrain/PTControl Example/PTControl_ALL_Speedgoat/New TC/TC R1/traction_controller ==
  max_torque : Inport
  dslip : Inport  Port=2
  enable_tc : Inport  Port=3
  Kp : Inport  Port=4
  Kd : Inport  Port=5
  Add : Sum  Inputs=+-
  Saturation Dynamic : simulink/Discontinuities/Saturation Dynamic  OutMin=[]  OutMax=[]  OutDataTypeStr=Inherit: Same as second input  OutDataType=fixdt(1, 16)  OutScaling=2^-10  DoSatur=off
  min_torque : Constant  Value=0
  traction_controller : Subsystem  TreatAsAtomicUnit=on
  delta_torque : Outport  VectorParamsAs1DForOutWhenUnconnected=off
  wires:
  Kd/1 -> traction_controller/4(Kd)
  enable_tc/1 -> traction_controller/2(enable_tc)
  Kp/1 -> traction_controller/3(Kp)
  traction_controller/1(delta_torque) -> Add/2
  dslip/1 -> traction_controller/1(dslip)
  Saturation Dynamic/1 -> delta_torque/1
  max_torque/1 -> Add/1, Saturation Dynamic/1
  min_torque/1 -> Saturation Dynamic/3
  Add/1 -> Saturation Dynamic/2

== system TorqueVect/CarMaker/IPG Vehicle/PowerTrain/PTControl Example/PTControl_ALL_Speedgoat/New TC/TC R2/traction_controller ==
  max_torque : Inport
  dslip : Inport  Port=2
  enable_tc : Inport  Port=3
  Kp : Inport  Port=4
  Kd : Inport  Port=5
  Add : Sum  Inputs=+-
  Saturation Dynamic : simulink/Discontinuities/Saturation Dynamic  OutMin=[]  OutMax=[]  OutDataTypeStr=Inherit: Same as second input  OutDataType=fixdt(1, 16)  OutScaling=2^-10  DoSatur=off
  min_torque : Constant  Value=0
  traction_controller : Subsystem  TreatAsAtomicUnit=on
  delta_torque : Outport  VectorParamsAs1DForOutWhenUnconnected=off
  wires:
  Kd/1 -> traction_controller/4(Kd)
  enable_tc/1 -> traction_controller/2(enable_tc)
  Kp/1 -> traction_controller/3(Kp)
  traction_controller/1(delta_torque) -> Add/2
  dslip/1 -> traction_controller/1(dslip)
  Saturation Dynamic/1 -> delta_torque/1
  max_torque/1 -> Add/1, Saturation Dynamic/1
  min_torque/1 -> Saturation Dynamic/3
  Add/1 -> Saturation Dynamic/2

== system TorqueVect/CarMaker/IPG Vehicle/PowerTrain/PTControl Example/PTControl_ALL_Speedgoat/New TC/TC R3/traction_controller ==
  max_torque : Inport
  dslip : Inport  Port=2
  enable_tc : Inport  Port=3
  Kp : Inport  Port=4
  Kd : Inport  Port=5
  Add : Sum  Inputs=+-
  Saturation Dynamic : simulink/Discontinuities/Saturation Dynamic  OutMin=[]  OutMax=[]  OutDataTypeStr=Inherit: Same as second input  OutDataType=fixdt(1, 16)  OutScaling=2^-10  DoSatur=off
  min_torque : Constant  Value=0
  traction_controller : Subsystem  TreatAsAtomicUnit=on
  delta_torque : Outport  VectorParamsAs1DForOutWhenUnconnected=off
  wires:
  Kd/1 -> traction_controller/4(Kd)
  enable_tc/1 -> traction_controller/2(enable_tc)
  Kp/1 -> traction_controller/3(Kp)
  traction_controller/1(delta_torque) -> Add/2
  dslip/1 -> traction_controller/1(dslip)
  Saturation Dynamic/1 -> delta_torque/1
  max_torque/1 -> Add/1, Saturation Dynamic/1
  min_torque/1 -> Saturation Dynamic/3
  Add/1 -> Saturation Dynamic/2

== system TorqueVect/CarMaker/IPG Vehicle/PowerTrain/PTControl Example/PTControl_ALL_Speedgoat/New TC/TC R4/traction_controller ==
  max_torque : Inport
  dslip : Inport  Port=2
  enable_tc : Inport  Port=3
  Kp : Inport  Port=4
  Kd : Inport  Port=5
  Add : Sum  Inputs=+-
  Saturation Dynamic : simulink/Discontinuities/Saturation Dynamic  OutMin=[]  OutMax=[]  OutDataTypeStr=Inherit: Same as second input  OutDataType=fixdt(1, 16)  OutScaling=2^-10  DoSatur=off
  min_torque : Constant  Value=0
  traction_controller : Subsystem  TreatAsAtomicUnit=on
  delta_torque : Outport  VectorParamsAs1DForOutWhenUnconnected=off
  wires:
  Kd/1 -> traction_controller/4(Kd)
  enable_tc/1 -> traction_controller/2(enable_tc)
  Kp/1 -> traction_controller/3(Kp)
  traction_controller/1(delta_torque) -> Add/2
  dslip/1 -> traction_controller/1(dslip)
  Saturation Dynamic/1 -> delta_torque/1
  max_torque/1 -> Add/1, Saturation Dynamic/1
  min_torque/1 -> Saturation Dynamic/3
  Add/1 -> Saturation Dynamic/2

== system TorqueVect/CarMaker/IPG Vehicle/PowerTrain/PTControl Example/PTControl_PC_MFE/New TC/TC R1/traction_controller ==
  max_torque : Inport
  dslip : Inport  Port=2
  enable_tc : Inport  Port=3
  Kp : Inport  Port=4
  Kd : Inport  Port=5
  Add : Sum  Inputs=+-
  Saturation Dynamic : simulink/Discontinuities/Saturation Dynamic  OutMin=[]  OutMax=[]  OutDataTypeStr=Inherit: Same as second input  OutDataType=fixdt(1, 16)  OutScaling=2^-10  DoSatur=off
  min_torque : Constant  Value=0
  traction_controller : Subsystem  TreatAsAtomicUnit=on
  delta_torque : Outport  VectorParamsAs1DForOutWhenUnconnected=off
  wires:
  Kd/1 -> traction_controller/4(Kd)
  enable_tc/1 -> traction_controller/2(enable_tc)
  Kp/1 -> traction_controller/3(Kp)
  traction_controller/1(delta_torque) -> Add/2
  dslip/1 -> traction_controller/1(dslip)
  Saturation Dynamic/1 -> delta_torque/1
  max_torque/1 -> Add/1, Saturation Dynamic/1
  min_torque/1 -> Saturation Dynamic/3
  Add/1 -> Saturation Dynamic/2

== system TorqueVect/CarMaker/IPG Vehicle/PowerTrain/PTControl Example/PTControl_PC_MFE/New TC/TC R2/traction_controller ==
  max_torque : Inport
  dslip : Inport  Port=2
  enable_tc : Inport  Port=3
  Kp : Inport  Port=4
  Kd : Inport  Port=5
  Add : Sum  Inputs=+-
  Saturation Dynamic : simulink/Discontinuities/Saturation Dynamic  OutMin=[]  OutMax=[]  OutDataTypeStr=Inherit: Same as second input  OutDataType=fixdt(1, 16)  OutScaling=2^-10  DoSatur=off
  min_torque : Constant  Value=0
  traction_controller : Subsystem  TreatAsAtomicUnit=on
  delta_torque : Outport  VectorParamsAs1DForOutWhenUnconnected=off
  wires:
  Kd/1 -> traction_controller/4(Kd)
  enable_tc/1 -> traction_controller/2(enable_tc)
  Kp/1 -> traction_controller/3(Kp)
  traction_controller/1(delta_torque) -> Add/2
  dslip/1 -> traction_controller/1(dslip)
  Saturation Dynamic/1 -> delta_torque/1
  max_torque/1 -> Add/1, Saturation Dynamic/1
  min_torque/1 -> Saturation Dynamic/3
  Add/1 -> Saturation Dynamic/2

== system TorqueVect/CarMaker/IPG Vehicle/PowerTrain/PTControl Example/PTControl_PC_MFE/New TC/TC R3/traction_controller ==
  max_torque : Inport
  dslip : Inport  Port=2
  enable_tc : Inport  Port=3
  Kp : Inport  Port=4
  Kd : Inport  Port=5
  Add : Sum  Inputs=+-
  Saturation Dynamic : simulink/Discontinuities/Saturation Dynamic  OutMin=[]  OutMax=[]  OutDataTypeStr=Inherit: Same as second input  OutDataType=fixdt(1, 16)  OutScaling=2^-10  DoSatur=off
  min_torque : Constant  Value=0
  traction_controller : Subsystem  TreatAsAtomicUnit=on
  delta_torque : Outport  VectorParamsAs1DForOutWhenUnconnected=off
  wires:
  Kd/1 -> traction_controller/4(Kd)
  enable_tc/1 -> traction_controller/2(enable_tc)
  Kp/1 -> traction_controller/3(Kp)
  traction_controller/1(delta_torque) -> Add/2
  dslip/1 -> traction_controller/1(dslip)
  Saturation Dynamic/1 -> delta_torque/1
  max_torque/1 -> Add/1, Saturation Dynamic/1
  min_torque/1 -> Saturation Dynamic/3
  Add/1 -> Saturation Dynamic/2

== system TorqueVect/CarMaker/IPG Vehicle/PowerTrain/PTControl Example/PTControl_PC_MFE/New TC/TC R4/traction_controller ==
  max_torque : Inport
  dslip : Inport  Port=2
  enable_tc : Inport  Port=3
  Kp : Inport  Port=4
  Kd : Inport  Port=5
  Add : Sum  Inputs=+-
  Saturation Dynamic : simulink/Discontinuities/Saturation Dynamic  OutMin=[]  OutMax=[]  OutDataTypeStr=Inherit: Same as second input  OutDataType=fixdt(1, 16)  OutScaling=2^-10  DoSatur=off
  min_torque : Constant  Value=0
  traction_controller : Subsystem  TreatAsAtomicUnit=on
  delta_torque : Outport  VectorParamsAs1DForOutWhenUnconnected=off
  wires:
  Kd/1 -> traction_controller/4(Kd)
  enable_tc/1 -> traction_controller/2(enable_tc)
  Kp/1 -> traction_controller/3(Kp)
  traction_controller/1(delta_torque) -> Add/2
  dslip/1 -> traction_controller/1(dslip)
  Saturation Dynamic/1 -> delta_torque/1
  max_torque/1 -> Add/1, Saturation Dynamic/1
  min_torque/1 -> Saturation Dynamic/3
  Add/1 -> Saturation Dynamic/2
